simulink model "full_adder"  (R2021a)
settings: Solver=VariableStepAuto  StartTime=0.0  StopTime=10.0  RelTol=1e-3
settings Model: Creator=kbhar  LastModifiedBy=kbhar

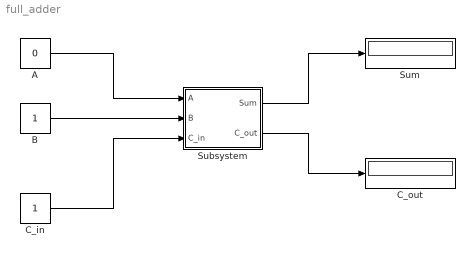
== system full_adder ==
  A : Constant  Value=0
  B : Constant
  C_in : Constant
  C_out : Display
  Subsystem : Subsystem
  Sum : Display
  wires:
  A/1 -> Subsystem/1(A)
  B/1 -> Subsystem/2(B)
  C_in/1 -> Subsystem/3(C_in)
  Subsystem/1(Sum) -> Sum/1
  Subsystem/2(C_out) -> C_out/1

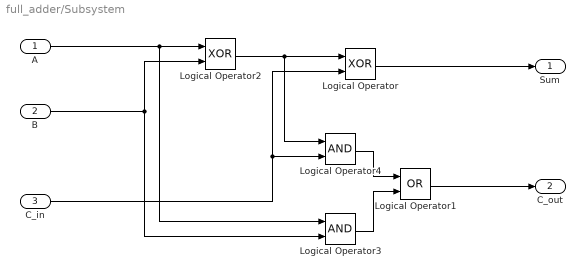
== system full_adder/Subsystem ==
  A : Inport
  B : Inport  Port=2
  C_in : Inport  Port=3
  Logical Operator : Logic  Operator=XOR  AllPortsSameDT=off  OutDataTypeStr=boolean
  Logical Operator1 : Logic  Operator=OR  AllPortsSameDT=off  OutDataTypeStr=boolean
  Logical Operator2 : Logic  Operator=XOR  AllPortsSameDT=off  OutDataTypeStr=boolean
  Logical Operator3 : Logic  AllPortsSameDT=off  OutDataTypeStr=boolean
  Logical Operator4 : Logic  AllPortsSameDT=off  OutDataTypeStr=boolean
  Sum : Outport
  C_out : Outport  Port=2
  wires:
  B/1 -> Logical Operator3/2, Logical Operator2/2
  A/1 -> Logical Operator3/1, Logical Operator2/1
  Logical Operator4/1 -> Logical Operator1/1
  Logical Operator/1 -> Sum/1
  Logical Operator2/1 -> Logical Operator4/1, Logical Operator/1
  C_in/1 -> Logical Operator4/2, Logical Operator/2
  Logical Operator3/1 -> Logical Operator1/2
  Logical Operator1/1 -> C_out/1
